simulink model "rotpentemplate_up_up"  (R2020b)
settings: Solver=ode45  StartTime=0.0  StopTime=100  RelTol=1e-3  EnableMultiTasking=on
values from neighbouring files (symbols this model uses):
  g01 = mean_data(2)    [MainScript_PID.m]    (also in calib_up_up.m)
  g02 = mean_data(3)    [MainScript_PID.m]    (also in calib_up_up.m)
  g11 = (mean_data(2)-mean_data(1))/pi    [MainScript_PID.m]    (also in calib_up_up.m)
  g12 = (mean_data(3)-mean_data(4))/pi    [MainScript_PID.m]    (also in calib_up_up.m)
  h = 0.01    [MainScript_PID.m]    (also in calib_up_up.m = 0.005)
  K = lqr(A, B, diag([10 20 200 110 10]), 350)    [calib_up_up.m]
undefined symbols (not defined in the file or in its folder): adingain, adinoffs, daoutgain, daoutoffs
libraries: dspsigops x2
settings Model: Creator=rbabuska  LastModifiedBy=cmatteo
settings DataIOCC: LimitDataPoints=on  SaveFormat=Array  ReturnWorkspaceOutputs=off  SignalLoggingName=sigsOut
settings OptimizationCC: BooleanDataType=off  ExpressionDepthLimit=2147483647  InitFltsAndDblsToZero=on  LifeSpan=inf
settings DebuggingCC: SaveWithParameterizedLinksMsg=none  SignalResolutionControl=TryResolveAllWithWarning  MultiTaskDSMMsg=warning  MultiTaskCondExecSysMsg=none  AllowSymbolicDim=off  StateNameClashWarn=warning  SFUnexpectedBacktrackingDiag=warning  SFNoUnconditionalDefaultTransitionDiag=warning  SFExecutionAtInitializationDiag=none  ArithmeticOperatorsInVariantConditions=warning
settings HardwareCC: ProdBitPerPointer=32  ProdBitPerSizeT=32  ProdBitPerPtrDiffT=32  ProdLargestAtomicFloat=None  ProdIntDivRoundTo=Undefined  ProdEndianess=Unspecified  ProdWordSize=32  ProdHWDeviceType=32-bit Generic  TargetUnknown=on
settings ModelReferenceCC: PropagateSignalLabelsOutOfModel=off
settings SFSimCC: SimUseLocalCustomCode=off  CustomCodeUndefinedFunction=UseInterfaceOnly
settings RTWCC: RTWUseLocalCustomCode=off
settings CodeAppCC: StateflowObjectComments=on
settings GRTTargetCC: TargetFcnLib=ansi_tfl_tmw.mat  TargetLangStandard=C89/C90 (ANSI)  CombineOutputUpdateFcns=off  GRTInterface=on
settings ConfigComp: CovMetricSettings=dw  CovSaveCumulativeToWorkspaceVar=on  CovSaveSingleToWorkspaceVar=on  CovExternalEMLEnable=off

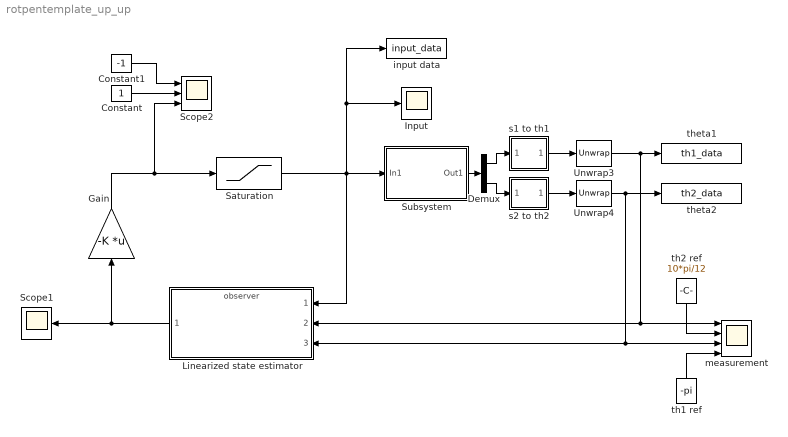
== system rotpentemplate_up_up ==
  Constant : Constant
  Constant1 : Constant  Value=-1
  Demux : Demux  Outputs=2
  Gain : Gain  Gain=-K  Multiplication=Matrix(K*u)
  Input : Scope
  Linearized state estimator : ModelReference  ModelNameDialog=observer.slx  SimulationMode=Normal  ModelReferenceVersion=1.10
  Saturation : Saturate  UpperLimit=1  LowerLimit=-1
  Scope1 : Scope
  Scope2 : Scope  NumInputPorts=3
  Subsystem : Subsystem
      mask Display: disp('Rotational\nPendulum')
  Unwrap3 : dspsigops/Unwrap  tol=pi  InputProcessing=Columns as channels (frame based)  running=off
  Unwrap4 : dspsigops/Unwrap  tol=pi  InputProcessing=Columns as channels (frame based)  running=off
  input data : ToWorkspace  VariableName=input_data  SaveFormat=Timeseries  SampleTime=h
  measurement : Scope  NumInputPorts=4
  s1 to th1 : Subsystem
  s2 to th2 : Subsystem
  th1 ref : Constant  Value=-pi
  th2 ref : Constant  Value=10*pi/12
  theta1 : ToWorkspace  VariableName=th1_data  SaveFormat=Timeseries  SampleTime=h
  theta2 : ToWorkspace  VariableName=th2_data  SaveFormat=Timeseries  SampleTime=h
  wires:
  Saturation/1 -> Linearized state estimator/1, Subsystem/1(In1), Input/1, input data/1
  Subsystem/1(Out1) -> Demux/1
  Demux/1 -> s1 to th1/1(v1)
  Demux/2 -> s2 to th2/1(v2)
  s1 to th1/1(th1) -> Unwrap3/1
  Unwrap3/1 -> measurement/1, Linearized state estimator/2, theta1/1
  s2 to th2/1(th2) -> Unwrap4/1
  Unwrap4/1 -> measurement/3, Linearized state estimator/3, theta2/1
  th1 ref/1 -> measurement/4
  th2 ref/1 -> measurement/2
  Linearized state estimator/1 -> Scope1/1, Gain/1
  Gain/1 -> Saturation/1, Scope2/3
  Constant/1 -> Scope2/2
  Constant1/1 -> Scope2/1

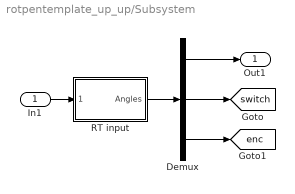
== system rotpentemplate_up_up/Subsystem ==
  In1 : Inport
  Demux : Demux  Outputs=[2 4 1]
  RT input : Subsystem  mask{Ts=h, channels=[6 7]}
      mask prompts: Ts "Sample time [s]:"; channels "Channels to read (e.g., [6 7])"
      mask init:
      | hwinit;
      | 
      | % initialize FPGA
      | fugihandle = fugiboard('Open', 'Pendulum1');
      | fugihandle.WatchdogTimeout = 0.5;
      | fugiboard('SetParams', fugihandle);
      | fugiboard('Write', fugihandle, 0, 0, 0, 0);  % dummy write to sync interface board
      | fugiboard('Write', fugihandle, 5, 1, 0, 0);  % reset position, activate relay
      | data = fugiboard('Read', fugihandle);        % get version info from FPGA
      | % model = bitshift(data(1), -5); 
      | % version = bitand(data(1), 31);
      | % disp(sprintf('FPGA setup %d, version %d', model, version)); % for the B&P it should say 1 1, or else there is a problem
      | fugiboard('Write', fugihandle, 0, 1, 0, 0);  % end reset
      | pause(0.1);                         % give relay some time to respond
      mask Display: disp('Rotational\nPendulum')
  Out1 : Outport
  tag scope: enc=global, switch=global
  wires:
  RT input/1(Angles) -> Demux/1
  Demux/1 -> Out1/1
  Demux/2 -> [switch]
  Demux/3 -> [enc]
  In1/1 -> RT input/1(Motors)

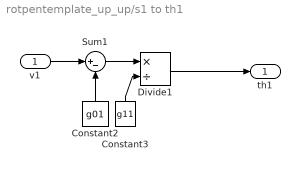
== system rotpentemplate_up_up/s1 to th1 ==
  v1 : Inport
  Constant2 : Constant  Value=g01
  Constant3 : Constant  Value=g11
  Divide1 : Product  Inputs=*/
  Sum1 : Sum  Inputs=|+-
  th1 : Outport
  wires:
  Constant2/1 -> Sum1/2
  Constant3/1 -> Divide1/2
  Divide1/1 -> th1/1
  Sum1/1 -> Divide1/1
  v1/1 -> Sum1/1

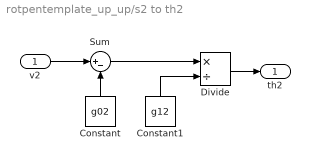
== system rotpentemplate_up_up/s2 to th2 ==
  v2 : Inport
  Constant : Constant  Value=g02
  Constant1 : Constant  Value=g12
  Divide : Product  Inputs=*/
  Sum : Sum  Inputs=|+-
  th2 : Outport
  wires:
  Constant1/1 -> Divide/2
  Divide/1 -> th2/1
  Constant/1 -> Sum/2
  Sum/1 -> Divide/1
  v2/1 -> Sum/1

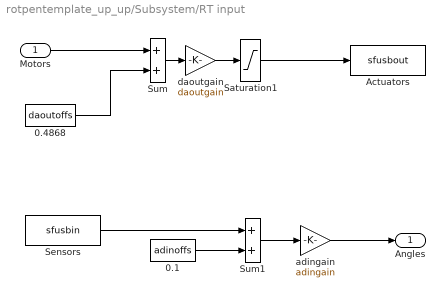
== system rotpentemplate_up_up/Subsystem/RT input ==
  Motors : Inport
  0.1 : Constant  Value=adinoffs
  0.4868 : Constant  Value=daoutoffs
  Actuators : S-Function  FunctionName=sfusbout  Parameters=Ts, fugihandle  SFunctionDeploymentMode=off  EnableBusSupport=off
  Saturation1 : Saturate  UpperLimit=10  LowerLimit=-10
  Sensors : S-Function  FunctionName=sfusbin  Parameters=Ts, fugihandle, channels  SFunctionDeploymentMode=off  EnableBusSupport=off
  Sum : Sum  InputSameDT=on  SaturateOnIntegerOverflow=on  OutDataTypeStr=Inherit: Same as first input
  Sum1 : Sum  InputSameDT=on  SaturateOnIntegerOverflow=on  OutDataTypeStr=Inherit: Same as first input
  adingain : Gain  Gain=adingain  SaturateOnIntegerOverflow=on  OutDataTypeStr=Inherit: Same as input  ParamDataTypeStr=Inherit: Same as input
  daoutgain : Gain  Gain=daoutgain  SaturateOnIntegerOverflow=on  OutDataTypeStr=Inherit: Same as input  ParamDataTypeStr=Inherit: Same as input
  Angles : Outport
  wires:
  Sum/1 -> daoutgain/1
  0.4868/1 -> Sum/2
  Motors/1 -> Sum/1
  Sum1/1 -> adingain/1
  0.1/1 -> Sum1/2
  adingain/1 -> Angles/1
  Saturation1/1 -> Actuators/1
  daoutgain/1 -> Saturation1/1
  Sensors/1 -> Sum1/1
